simulink library "LIB_OutputsProcessing"  (R2018b)
settings: Solver=VariableStepAuto  StartTime=0.0  StopTime=10.0  RelTol=1e-3
undefined symbols (not defined in the file or in its folder): eActuators, NActuatorActive, nBlowerCmdMax, nBlowerCmdTestInactive, rActuatorCmdMaxRatio, rBlowerPwmMinSat, rValveCmdTestInactive
libraries: simulink x5, RespiratorCtrlLib x3
settings Model: Creator=BRAUL  LastModifiedBy=BRAUL

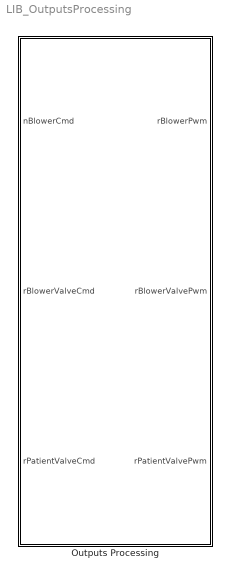
== system LIB_OutputsProcessing ==
  Outputs Processing : Subsystem
      settings: AttributesFormatString=%<ReferenceBlock>

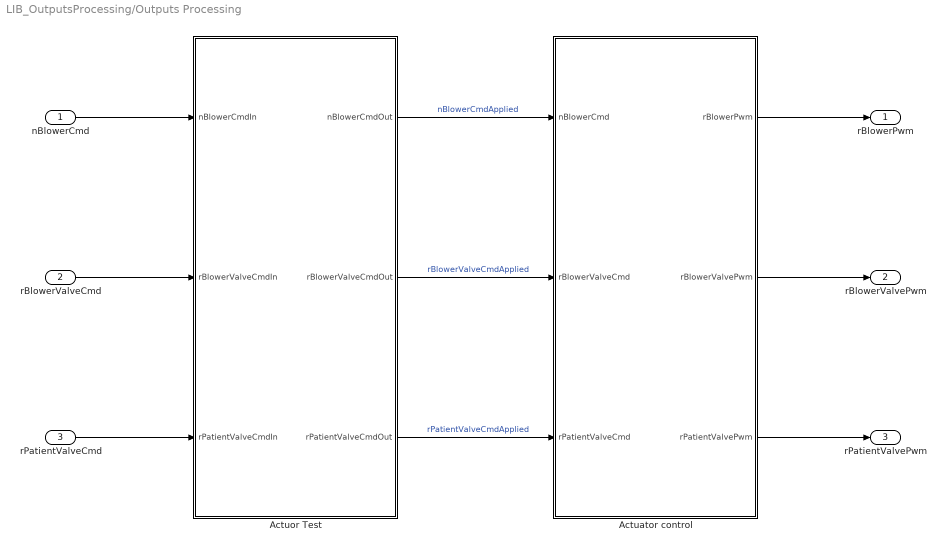
== system LIB_OutputsProcessing/Outputs Processing ==
  nBlowerCmd : Inport
  rBlowerValveCmd : Inport  Port=2
  rPatientValveCmd : Inport  Port=3
  Actuator control : Subsystem  Priority=1  TreatAsAtomicUnit=on
      settings: AttributesFormatString=Priority %<Priority>
  Actuor Test : Subsystem  Priority=0  TreatAsAtomicUnit=on
      settings: AttributesFormatString=Priority %<Priority>
  rBlowerPwm : Outport
  rBlowerValvePwm : Outport  Port=2
  rPatientValvePwm : Outport  Port=3
  wires:
  Actuor Test/3(rPatientValveCmdOut) -> Actuator control/3(rPatientValveCmd)  "rPatientValveCmdApplied"
  Actuor Test/2(rBlowerValveCmdOut) -> Actuator control/2(rBlowerValveCmd)  "rBlowerValveCmdApplied"
  Actuor Test/1(nBlowerCmdOut) -> Actuator control/1(nBlowerCmd)  "nBlowerCmdApplied"
  rPatientValveCmd/1 -> Actuor Test/3(rPatientValveCmdIn)
  rBlowerValveCmd/1 -> Actuor Test/2(rBlowerValveCmdIn)
  nBlowerCmd/1 -> Actuor Test/1(nBlowerCmdIn)
  Actuator control/3(rPatientValvePwm) -> rPatientValvePwm/1
  Actuator control/2(rBlowerValvePwm) -> rBlowerValvePwm/1
  Actuator control/1(rBlowerPwm) -> rBlowerPwm/1

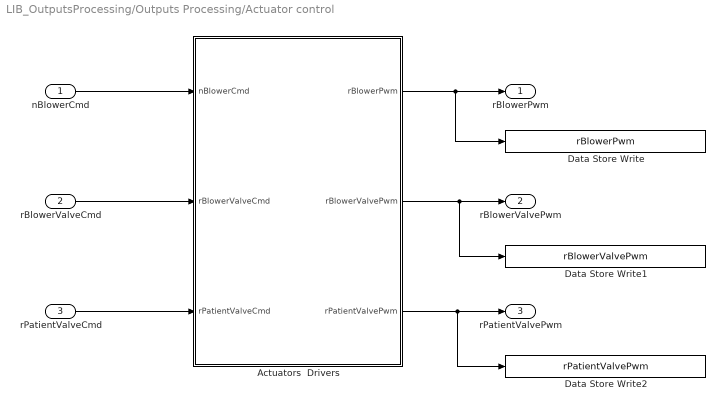
== system LIB_OutputsProcessing/Outputs Processing/Actuator control ==
  nBlowerCmd : Inport  OutDataTypeStr=single
  rBlowerValveCmd : Inport  Port=2  OutDataTypeStr=single
  rPatientValveCmd : Inport  Port=3  OutDataTypeStr=single
  Actuators  Drivers : Subsystem
  Data Store Write : DataStoreWrite  DataStoreName=rBlowerPwm
  Data Store Write1 : DataStoreWrite  DataStoreName=rBlowerValvePwm
  Data Store Write2 : DataStoreWrite  DataStoreName=rPatientValvePwm
  rBlowerPwm : Outport
  rBlowerValvePwm : Outport  Port=2
  rPatientValvePwm : Outport  Port=3
  wires:
  nBlowerCmd/1 -> Actuators  Drivers/1(nBlowerCmd)
  rBlowerValveCmd/1 -> Actuators  Drivers/2(rBlowerValveCmd)
  rPatientValveCmd/1 -> Actuators  Drivers/3(rPatientValveCmd)
  Actuators  Drivers/1(rBlowerPwm) -> rBlowerPwm/1, Data Store Write/1
  Actuators  Drivers/2(rBlowerValvePwm) -> rBlowerValvePwm/1, Data Store Write1/1
  Actuators  Drivers/3(rPatientValvePwm) -> rPatientValvePwm/1, Data Store Write2/1

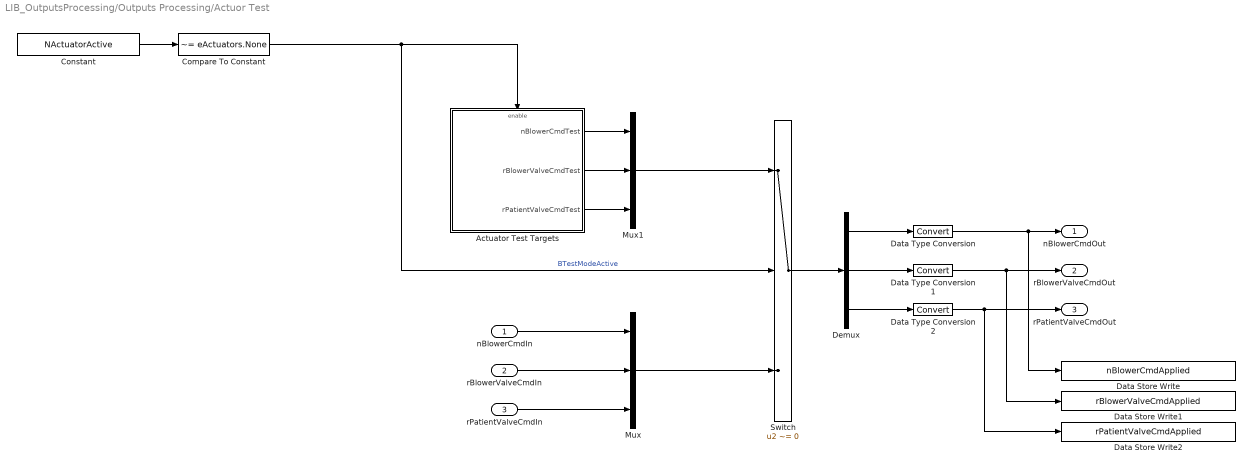
== system LIB_OutputsProcessing/Outputs Processing/Actuor Test ==
  nBlowerCmdIn : Inport  OutDataTypeStr=single
  rBlowerValveCmdIn : Inport  Port=2  OutDataTypeStr=single
  rPatientValveCmdIn : Inport  Port=3  OutDataTypeStr=single
  Actuator Test Targets : Subsystem
  Compare To Constant : simulink/Logic and Bit Operations/Compare To Constant  relop=~=  const=eActuators.None  OutDataTypeStr=boolean
  Constant : Constant  Value=NActuatorActive  OutDataTypeStr=Enum: eActuators
  Data Store Write : DataStoreWrite  DataStoreName=nBlowerCmdApplied
  Data Store Write1 : DataStoreWrite  DataStoreName=rBlowerValveCmdApplied
  Data Store Write2 : DataStoreWrite  DataStoreName=rPatientValveCmdApplied
  Data Type Conversion : DataTypeConversion
  Data Type Conversion1 : DataTypeConversion
  Data Type Conversion2 : DataTypeConversion
  Demux : Demux  Outputs=3
  Mux : Mux  Inputs=3
  Mux1 : Mux  Inputs=3
  Switch : Switch  Criteria=u2 ~= 0
  nBlowerCmdOut : Outport
  rBlowerValveCmdOut : Outport  Port=2
  rPatientValveCmdOut : Outport  Port=3
  wires:
  Compare To Constant/1 -> Switch/2, Actuator Test Targets/Enable  "BTestModeActive"
  Constant/1 -> Compare To Constant/1
  Data Type Conversion2/1 -> rPatientValveCmdOut/1, Data Store Write2/1
  Data Type Conversion1/1 -> rBlowerValveCmdOut/1, Data Store Write1/1
  Data Type Conversion/1 -> nBlowerCmdOut/1, Data Store Write/1
  Switch/1 -> Demux/1
  Mux1/1 -> Switch/1
  Actuator Test Targets/3(rPatientValveCmdTest) -> Mux1/3
  Actuator Test Targets/2(rBlowerValveCmdTest) -> Mux1/2
  Actuator Test Targets/1(nBlowerCmdTest) -> Mux1/1
  Demux/3 -> Data Type Conversion2/1
  Demux/2 -> Data Type Conversion1/1
  Demux/1 -> Data Type Conversion/1
  rPatientValveCmdIn/1 -> Mux/3
  rBlowerValveCmdIn/1 -> Mux/2
  nBlowerCmdIn/1 -> Mux/1
  Mux/1 -> Switch/3

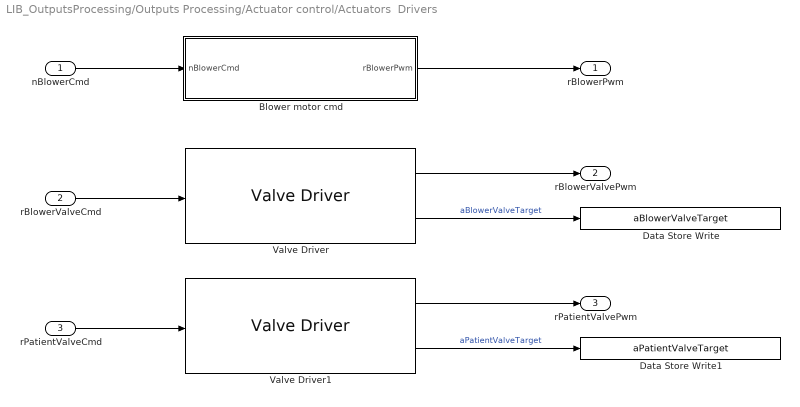
== system LIB_OutputsProcessing/Outputs Processing/Actuator control/Actuators  Drivers ==
  nBlowerCmd : Inport  OutDataTypeStr=single
  rBlowerValveCmd : Inport  Port=2  OutDataTypeStr=single
  rPatientValveCmd : Inport  Port=3  OutDataTypeStr=single
  Blower motor cmd : Subsystem
  Data Store Write : DataStoreWrite  DataStoreName=aBlowerValveTarget
  Data Store Write1 : DataStoreWrite  DataStoreName=aPatientValveTarget
  Valve Driver : RespiratorCtrlLib/Outputs/Valve Driver  outputName=Blower Valve  closeAngle=aValveFullClose  openAngle=aValveFullOpen  zeroDegPwm=rPwmZeroDeg  posPwmMax=aValvePwm100  gainPos=NaN  offsetPos=NaN  gainPwm=NaN  offsetPwm=0
  Valve Driver1 : RespiratorCtrlLib/Outputs/Valve Driver  outputName=Patient Valve  closeAngle=aValveFullClose  openAngle=aValveFullOpen  zeroDegPwm=rPwmZeroDeg  posPwmMax=aValvePwm100  gainPos=NaN  offsetPos=NaN  gainPwm=NaN  offsetPwm=0
  rBlowerPwm : Outport
  rBlowerValvePwm : Outport  Port=2
  rPatientValvePwm : Outport  Port=3
  wires:
  Valve Driver1/2 -> Data Store Write1/1  "aPatientValveTarget"
  Valve Driver/2 -> Data Store Write/1  "aBlowerValveTarget"
  rPatientValveCmd/1 -> Valve Driver1/1
  Blower motor cmd/1(rBlowerPwm) -> rBlowerPwm/1
  Valve Driver/1 -> rBlowerValvePwm/1
  rBlowerValveCmd/1 -> Valve Driver/1
  Valve Driver1/1 -> rPatientValvePwm/1
  nBlowerCmd/1 -> Blower motor cmd/1(nBlowerCmd)

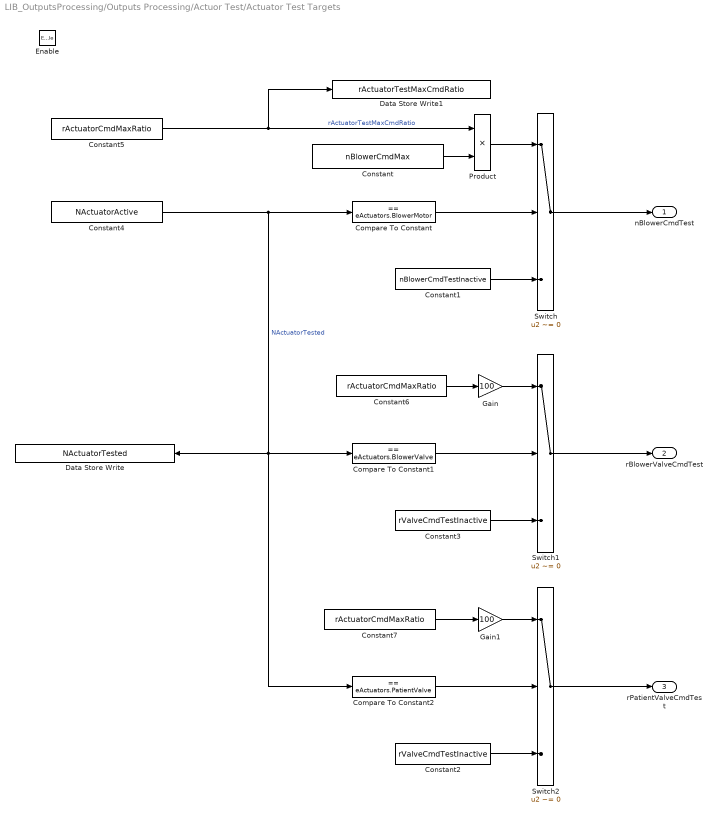
== system LIB_OutputsProcessing/Outputs Processing/Actuor Test/Actuator Test Targets ==
  Enable : EnablePort  StatesWhenEnabling=reset
  Compare To Constant : simulink/Logic and Bit Operations/Compare To Constant  relop===  const=eActuators.BlowerMotor  OutDataTypeStr=boolean
  Compare To Constant1 : simulink/Logic and Bit Operations/Compare To Constant  relop===  const=eActuators.BlowerValve  OutDataTypeStr=boolean
  Compare To Constant2 : simulink/Logic and Bit Operations/Compare To Constant  relop===  const=eActuators.PatientValve  OutDataTypeStr=boolean
  Constant : Constant  Value=nBlowerCmdMax
  Constant1 : Constant  Value=nBlowerCmdTestInactive
  Constant2 : Constant  Value=rValveCmdTestInactive
  Constant3 : Constant  Value=rValveCmdTestInactive
  Constant4 : Constant  Value=NActuatorActive  OutDataTypeStr=Enum: eActuators
  Constant5 : Constant  Value=rActuatorCmdMaxRatio  OutDataTypeStr=single
  Constant6 : Constant  Value=rActuatorCmdMaxRatio  OutDataTypeStr=single
  Constant7 : Constant  Value=rActuatorCmdMaxRatio  OutDataTypeStr=single
  Data Store Write : DataStoreWrite  DataStoreName=NActuatorTested
  Data Store Write1 : DataStoreWrite  DataStoreName=rActuatorTestMaxCmdRatio
  Gain : Gain  Gain=100
  Gain1 : Gain  Gain=100
  Product : Product
  Switch : Switch  Criteria=u2 ~= 0
  Switch1 : Switch  Criteria=u2 ~= 0
  Switch2 : Switch  Criteria=u2 ~= 0
  nBlowerCmdTest : Outport  OutputWhenDisabled=reset  InitialOutput=nBlowerCmdTestInactive
  rBlowerValveCmdTest : Outport  Port=2  OutputWhenDisabled=reset  InitialOutput=rValveCmdTestInactive
  rPatientValveCmdTest : Outport  Port=3  OutputWhenDisabled=reset  InitialOutput=rValveCmdTestInactive
  wires:
  Gain1/1 -> Switch2/1
  Constant7/1 -> Gain1/1
  Gain/1 -> Switch1/1
  Constant6/1 -> Gain/1
  Constant3/1 -> Switch1/3
  Constant2/1 -> Switch2/3
  Product/1 -> Switch/1
  Constant5/1 -> Product/1, Data Store Write1/1  "rActuatorTestMaxCmdRatio"
  Constant/1 -> Product/2
  Switch2/1 -> rPatientValveCmdTest/1
  Compare To Constant2/1 -> Switch2/2
  Switch1/1 -> rBlowerValveCmdTest/1
  Compare To Constant1/1 -> Switch1/2
  Constant4/1 -> Compare To Constant/1, Compare To Constant1/1, Compare To Constant2/1, Data Store Write/1  "NActuatorTested"
  Switch/1 -> nBlowerCmdTest/1
  Constant1/1 -> Switch/3
  Compare To Constant/1 -> Switch/2

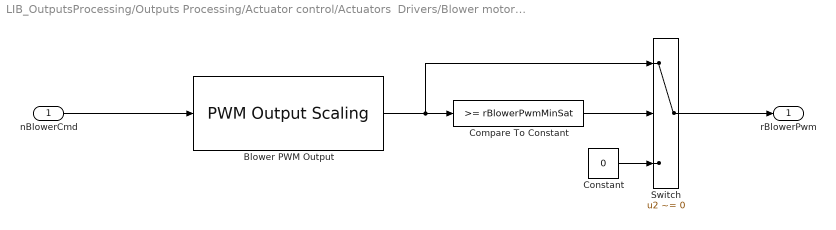
== system LIB_OutputsProcessing/Outputs Processing/Actuator control/Actuators  Drivers/Blower motor cmd ==
  nBlowerCmd : Inport
  Blower PWM Output : RespiratorCtrlLib/Outputs/PWM Output Scaling  outputName=Blower  physicMin=nBlowerTargetMin  physicMax=nBlowerTargetMax  gain=0  offset=0
  Compare To Constant : simulink/Logic and Bit Operations/Compare To Constant  relop=>=  const=rBlowerPwmMinSat  OutDataTypeStr=boolean
  Constant : Constant  Value=0  OutDataTypeStr=single
  Switch : Switch  Criteria=u2 ~= 0
  rBlowerPwm : Outport
  wires:
  nBlowerCmd/1 -> Blower PWM Output/1
  Blower PWM Output/1 -> Switch/1, Compare To Constant/1
  Compare To Constant/1 -> Switch/2
  Constant/1 -> Switch/3
  Switch/1 -> rBlowerPwm/1
